simulink model "single_phase_inverter_rpid"  (R2019b)
settings: Solver=VariableStepAuto  StartTime=0.0  StopTime=simlength  RelTol=1e-3
values from neighbouring files (symbols this model uses):
  A = [-R1/L1 0 -1/L1;      0 -R2/L2 1/L2;      1/C1 -1/C1 0]    [inverter_singlephase.m]    (also in inverter_singlephase_rpi.m)
  Aed = eye(4) + A*Ts+ A^2*Ts^2/2 + A^3*Ts^3/factorial(3)+ A^3*Ts^4/factorial(4)    [inverter_singlephase.m]    (also in inverter_singlephase_rpi.m = eye(5) + Ae*Ts + Ae^2*Ts^2/2 + Ae^3*Ts^3/factorial(3)+ Ae^3*)
  Aresd = [cos(w0*Ts) sin(w0*Ts)/w0; -w0*sin(w0*Ts) cos(w0*Ts)]    [inverter_singlephase_rpi.m]
  B = [1/L1 0 0]'    [inverter_singlephase.m]    (also in inverter_singlephase_rpi.m)
  Bed = B*Ts + A*B*Ts^2/2 + A^2*B*Ts^3/factorial(3) + A^3*B*Ts^4/factorial(4)     + A^4*B*Ts^5/factorial(5)    [inverter_singlephase.m]    (also in inverter_singlephase_rpi.m = Be*Ts + Ae*Be*Ts^2/2 + Ae^2*Be*Ts^3/factorial(3) + Ae^3*Be*T)
  Bresd = [(1-cos(w0*Ts))/w0^2 sin(w0*Ts)/w0]'    [inverter_singlephase_rpi.m]
  C = [1 0 0; 0 0 1]    [inverter_singlephase.m]    (also in inverter_singlephase_rpi.m)
  Ce = [1 0 0 0 0; 0 0 1 0 0]    [inverter_singlephase.m]    (also in inverter_singlephase_rpi.m)
  Cres = [0 1]    [inverter_singlephase_rpi.m]
  d = 3.5e-1    (= 0.35)    [inverter_singlephase.m]    (also in inverter_singlephase_rpi.m)
  E = [0 -1/L2 0]'    [inverter_singlephase.m]    (also in inverter_singlephase_rpi.m)
  ki = 35    [inverter_singlephase.m]    (also in inverter_singlephase_rpi.m)
  kp = 1    [inverter_singlephase.m]    (also in inverter_singlephase_rpi.m)
  Led = place(Aed',Ce',zp)'    [inverter_singlephase_rpi.m]
  simlength = 0.1    [inverter_singlephase.m]    (also in inverter_singlephase_rpi.m)
  Tc = 1e-5    (= 1e-05)    [inverter_singlephase_rpi.m]
  Ts = 1e-4    (= 0.0001)    [inverter_singlephase.m]    (also in inverter_singlephase_rpi.m)
  w = 5*w0    (= 1570.79632679)    [inverter_singlephase.m]    (also in inverter_singlephase_rpi.m)
  w0 = 2*pi*50    (= 314.159265359)    [inverter_singlephase.m]    (also in inverter_singlephase_rpi.m)
settings Model: Creator=dbagn  LastModifiedBy=dbagn
settings DataIOCC: ReturnWorkspaceOutputs=off

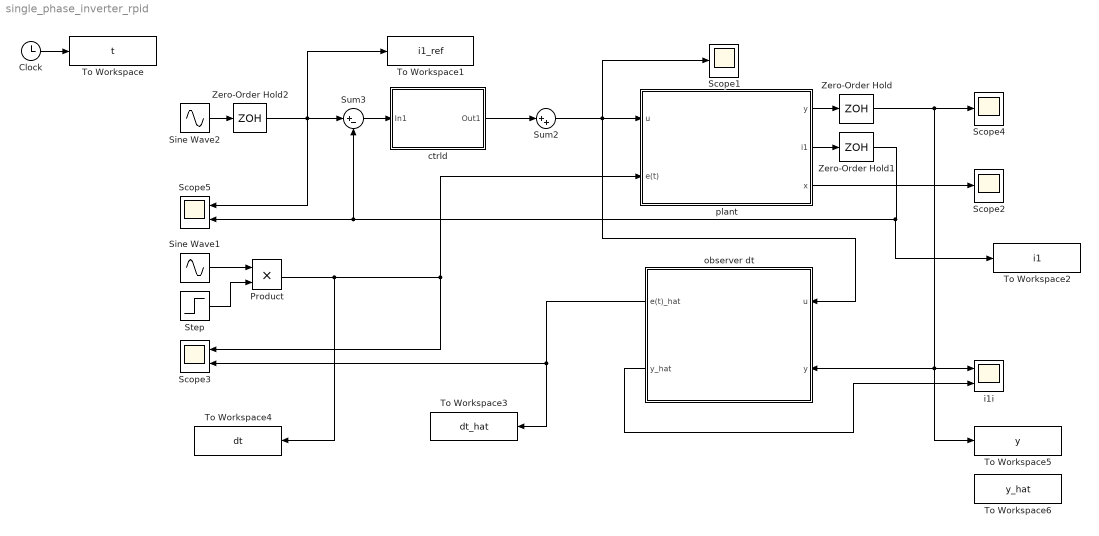
== system single_phase_inverter_rpid ==
  Clock : Clock
  Product : Product
  Scope1 : Scope
  Scope2 : Scope
  Scope3 : Scope  NumInputPorts=2
  Scope4 : Scope
  Scope5 : Scope  NumInputPorts=2
  Sine Wave1 : Sin  Amplitude=d  Frequency=w  SampleTime=0
  Sine Wave2 : Sin  Frequency=w0  SampleTime=0
  Step : Step  Time=simlength/2  SampleTime=0
  Sum2 : Sum  Inputs=|++
  Sum3 : Sum  Inputs=|+-
  To Workspace : ToWorkspace  VariableName=t  SampleTime=Tc
      settings: MaxDataPoints=Nc
  To Workspace1 : ToWorkspace  VariableName=i1_ref  SampleTime=Tc
      settings: MaxDataPoints=Nc
  To Workspace2 : ToWorkspace  VariableName=i1  SampleTime=Tc
      settings: MaxDataPoints=Nc
  To Workspace3 : ToWorkspace  VariableName=dt_hat  SampleTime=Tc
      settings: MaxDataPoints=Nc
  To Workspace4 : ToWorkspace  VariableName=dt  SampleTime=Tc
      settings: MaxDataPoints=Nc
  To Workspace5 : ToWorkspace  VariableName=y  SampleTime=Tc
      settings: MaxDataPoints=Nc
  To Workspace6 : ToWorkspace  VariableName=y_hat  SampleTime=Tc
      settings: MaxDataPoints=Nc
  Zero-Order Hold : ZeroOrderHold  SampleTime=Ts
  Zero-Order Hold1 : ZeroOrderHold  SampleTime=Ts
  Zero-Order Hold2 : ZeroOrderHold  SampleTime=Ts
  ctrld : Subsystem
  i1i : Scope  NumInputPorts=2
  observer dt : Subsystem
  "plant " : Subsystem
  wires:
  observer dt/2(y_hat) -> i1i/2
  "plant "/1(y) -> Zero-Order Hold/1
  Product/1 -> To Workspace4/1, Scope3/1, "plant "/2(e(t))
  Sine Wave2/1 -> Zero-Order Hold2/1
  ctrld/1(Out1) -> Sum2/1
  Sum2/1 -> observer dt/1(u), "plant "/1(u), Scope1/1
  "plant "/2(i1) -> Zero-Order Hold1/1
  "plant "/3(x) -> Scope2/1
  Sum3/1 -> ctrld/1(In1)
  observer dt/1(e(t)_hat) -> To Workspace3/1, Scope3/2
  Zero-Order Hold/1 -> To Workspace5/1, observer dt/2(y), i1i/1, Scope4/1
  Zero-Order Hold1/1 -> To Workspace2/1, Sum3/2, Scope5/2
  Zero-Order Hold2/1 -> To Workspace1/1, Sum3/1, Scope5/1
  Sine Wave1/1 -> Product/1
  Step/1 -> Product/2
  Clock/1 -> To Workspace/1

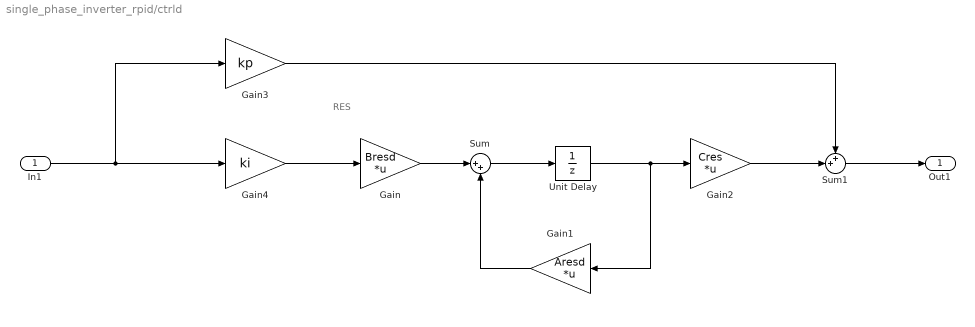
== system single_phase_inverter_rpid/ctrld ==
  note: RES
  In1 : Inport
  Gain : Gain  Gain=Bresd  Multiplication=Matrix(K*u)
  Gain1 : Gain  Gain=Aresd  Multiplication=Matrix(K*u)
  Gain2 : Gain  Gain=Cres  Multiplication=Matrix(K*u)
  Gain3 : Gain  Gain=kp
  Gain4 : Gain  Gain=ki
  Sum : Sum  Inputs=|++
  Sum1 : Sum  Inputs=++|
  Unit Delay : UnitDelay  SampleTime=Ts  HasFrameUpgradeWarning=on
  Out1 : Outport
  wires:
  In1/1 -> Gain4/1, Gain3/1
  Sum/1 -> Unit Delay/1
  Gain/1 -> Sum/1
  Gain1/1 -> Sum/2
  Unit Delay/1 -> Gain2/1, Gain1/1
  Gain4/1 -> Gain/1
  Gain2/1 -> Sum1/2
  Sum1/1 -> Out1/1
  Gain3/1 -> Sum1/1

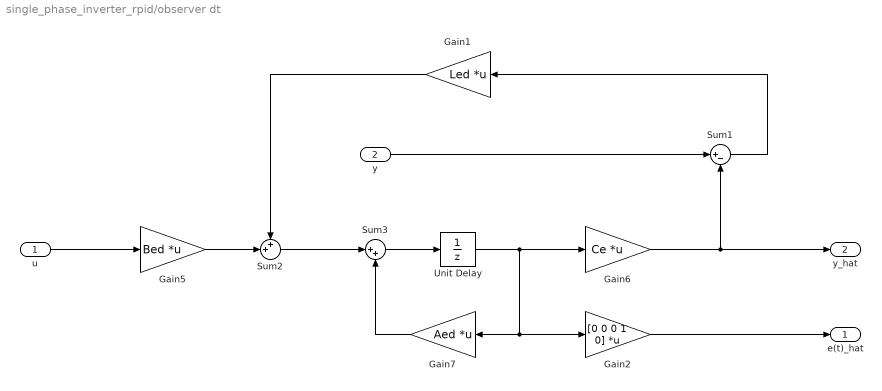
== system single_phase_inverter_rpid/observer dt ==
  u : Inport
  y : Inport  Port=2
  Gain1 : Gain  Gain=Led  Multiplication=Matrix(K*u)
  Gain2 : Gain  Gain=[0 0 0 1 0]  Multiplication=Matrix(K*u)
  Gain5 : Gain  Gain=Bed  Multiplication=Matrix(K*u)
  Gain6 : Gain  Gain=Ce  Multiplication=Matrix(K*u)
  Gain7 : Gain  Gain=Aed  Multiplication=Matrix(K*u)
  Sum1 : Sum  Inputs=|+-
  Sum2 : Sum  Inputs=++|
  Sum3 : Sum  Inputs=|++
  Unit Delay : UnitDelay  SampleTime=Ts  HasFrameUpgradeWarning=on
  e(t)_hat : Outport
  y_hat : Outport  Port=2
  wires:
  Sum2/1 -> Sum3/1
  Gain7/1 -> Sum3/2
  Gain6/1 -> y_hat/1, Sum1/2
  Sum1/1 -> Gain1/1
  u/1 -> Gain5/1
  Gain1/1 -> Sum2/1
  Gain5/1 -> Sum2/2
  y/1 -> Sum1/1
  Gain2/1 -> e(t)_hat/1
  Sum3/1 -> Unit Delay/1
  Unit Delay/1 -> Gain2/1, Gain7/1, Gain6/1

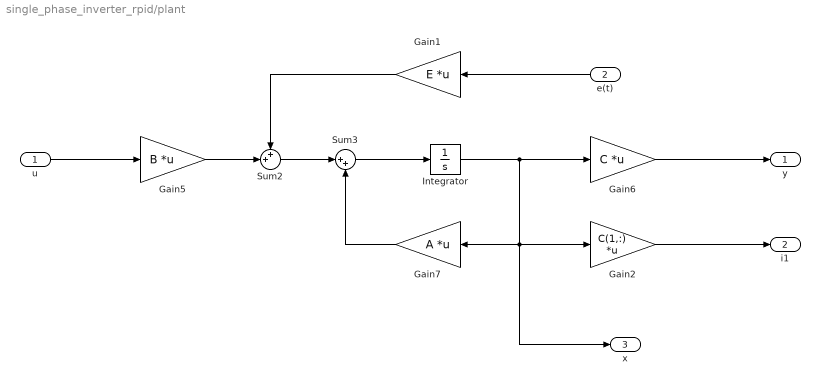
== system single_phase_inverter_rpid/plant  ==
  u : Inport
  e(t) : Inport  Port=2
  Gain1 : Gain  Gain=E  Multiplication=Matrix(K*u)
  Gain2 : Gain  Gain=C(1,:)  Multiplication=Matrix(K*u)
  Gain5 : Gain  Gain=B  Multiplication=Matrix(K*u)
  Gain6 : Gain  Gain=C  Multiplication=Matrix(K*u)
  Gain7 : Gain  Gain=A  Multiplication=Matrix(K*u)
  Integrator : Integrator
  Sum2 : Sum  Inputs=++|
  Sum3 : Sum  Inputs=|++
  y : Outport
  i1 : Outport  Port=2
  x : Outport  Port=3
  wires:
  Sum3/1 -> Integrator/1
  Gain5/1 -> Sum2/2
  Gain1/1 -> Sum2/1
  Gain7/1 -> Sum3/2
  u/1 -> Gain5/1
  Sum2/1 -> Sum3/1
  Gain6/1 -> y/1
  e(t)/1 -> Gain1/1
  Integrator/1 -> x/1, Gain2/1, Gain7/1, Gain6/1
  Gain2/1 -> i1/1
